simulink model "r_PGU"  (R2018b)
settings: Solver=VariableStepAuto  StartTime=0.0  StopTime=10.0  RelTol=1e-3
undefined symbols (not defined in the file): G_bPF, I_bPF, r_bPGU
settings Model: Creator=rache  LastModifiedBy=rache

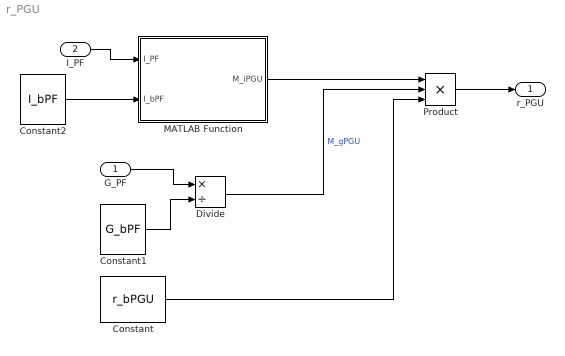
== system r_PGU ==
  G_PF : Inport
  I_PF : Inport  Port=2
  Constant : Constant  Value=r_bPGU
  Constant1 : Constant  Value=G_bPF
  Constant2 : Constant  Value=I_bPF
  Divide : Product  Inputs=*/
  MATLAB Function : MATLAB Function  TreatAsAtomicUnit=on
  Product : Product  Inputs=3
  r_PGU : Outport
  wires:
  G_PF/1 -> Divide/1
  Constant1/1 -> Divide/2
  Constant2/1 -> MATLAB Function/2(I_bPF)
  I_PF/1 -> MATLAB Function/1(I_PF)
  MATLAB Function/1(M_iPGU) -> Product/1
  Divide/1 -> Product/2  "M_gPGU"
  Constant/1 -> Product/3
  Product/1 -> r_PGU/1

== matlab function r_PGU/MATLAB Function ==
  data: I_PF input; M_iPGU output; I_bPF input
function M_iPGU = fcn(I_PF, I_bPF)

M_iPGU = 7.03 + 6.52*(tanh(0.338*(I_PF/I_bPF - 5.82)));
